simulink model "sim_fake"  (Simulink 8.4)
settings: Solver=ode23s  StartTime=0.0  StopTime=max(time)  FixedStep=0.0001  RelTol=1e-3
values from neighbouring files (symbols this model uses):
  CTRL = ctrl_d(7)    [step4_simulation.m]    (also in step5_yaml.m = ctrl_d(i))
  PLANT = model.chip    [step2_design_controller.m]    (also in step3_check_performance.m = model.combo; step4_simulation.m = model.combo; step99_validation.m = model.combo)
settings Model: Creator=yh3wong  LastModifiedBy=yh3wong
settings DataIOCC: SignalLoggingSaveFormat=Dataset
settings OptimizationCC: ExpressionDepthLimit=128
settings DebuggingCC: UnderspecifiedInitializationDetection=Simplified  MergeDetectMultiDrivingBlocksExec=error  FcnCallInpInsideContextMsg=EnableAllAsError  StateNameClashWarn=none
settings GRTTargetCC: CombineOutputUpdateFcns=on  GRTInterface=off

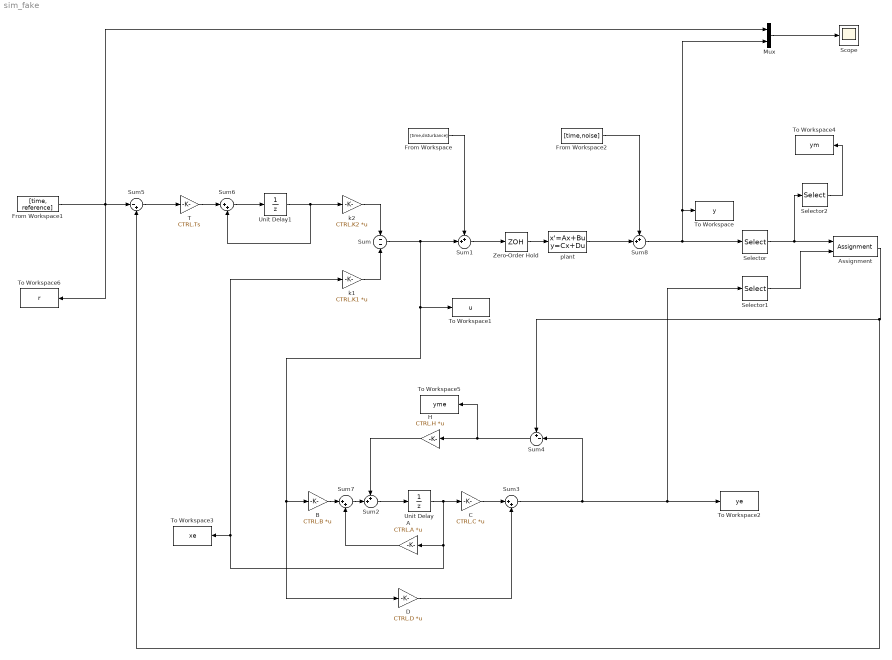
== system sim_fake ==
  A : Gain  Gain=CTRL.A  Multiplication=Matrix(K*u)  SampleTime=CTRL.Ts
  Assignment : Assignment  DiagnosticForDimensions=Warning  SampleTime=CTRL.Ts  Indices=FAKE
  B : Gain  Gain=CTRL.B  Multiplication=Matrix(K*u)  SampleTime=CTRL.Ts
  C : Gain  Gain=CTRL.C  Multiplication=Matrix(K*u)  SampleTime=CTRL.Ts
  D : Gain  Gain=CTRL.D  Multiplication=Matrix(K*u)  SampleTime=CTRL.Ts
  From Workspace : FromWorkspace  VariableName=[time,disturbance]  SampleTime=CTRL.Ts  Interpolate=off  OutputAfterFinalValue=Holding final value
  From Workspace1 : FromWorkspace  VariableName=[time, reference]  SampleTime=CTRL.Ts  Interpolate=off  OutputAfterFinalValue=Holding final value
  From Workspace2 : FromWorkspace  VariableName=[time,noise]  OutputAfterFinalValue=Holding final value
  H : Gain  Gain=CTRL.H  Multiplication=Matrix(K*u)  SampleTime=CTRL.Ts
  Mux : Mux  Inputs=2
  Scope : Scope
      settings: YMin=-150  YMax=200
  Selector : Selector  InputPortWidth=length(PLANT.output)  Indices=CTRL.channel_idx
  Selector1 : Selector  InputPortWidth=length(CTRL.output)  Indices=FAKE
  Selector2 : Selector  InputPortWidth=length(CTRL.output)  Indices=REAL
  Sum : Sum  Inputs=-|-  SampleTime=CTRL.Ts
  Sum1 : Sum  Inputs=++|  SampleTime=CTRL.Ts
  Sum2 : Sum  Inputs=++|  SampleTime=CTRL.Ts
  Sum3 : Sum  Inputs=|++  SampleTime=CTRL.Ts
  Sum4 : Sum  Inputs=+-|  SampleTime=CTRL.Ts
  Sum5 : Sum  Inputs=|-+  SampleTime=CTRL.Ts
  Sum6 : Sum  Inputs=|++  SampleTime=CTRL.Ts
  Sum7 : Sum  Inputs=|++  SampleTime=CTRL.Ts
  Sum8 : Sum  Inputs=++|
  T : Gain  Gain=CTRL.Ts  SampleTime=CTRL.Ts
  To Workspace : ToWorkspace  VariableName=y  SaveFormat=Structure With Time  SampleTime=-1
  To Workspace1 : ToWorkspace  VariableName=u  SaveFormat=Structure With Time  SampleTime=CTRL.Ts
  To Workspace2 : ToWorkspace  VariableName=ye  SaveFormat=Structure With Time  SampleTime=CTRL.Ts
  To Workspace3 : ToWorkspace  VariableName=xe  SaveFormat=Structure With Time  SampleTime=CTRL.Ts
  To Workspace4 : ToWorkspace  VariableName=ym  SaveFormat=Structure With Time  SampleTime=-1
  To Workspace5 : ToWorkspace  VariableName=yme  SaveFormat=Structure With Time  SampleTime=CTRL.Ts
  To Workspace6 : ToWorkspace  VariableName=r  SaveFormat=Structure With Time  SampleTime=CTRL.Ts
  Unit Delay : UnitDelay  SampleTime=CTRL.Ts
  Unit Delay1 : UnitDelay  SampleTime=CTRL.Ts
  Zero-Order Hold : ZeroOrderHold  SampleTime=CTRL.Ts
  "k1 " : Gain  Gain=CTRL.K1  Multiplication=Matrix(K*u)  SampleTime=CTRL.Ts
  k2 : Gain  Gain=CTRL.K2  Multiplication=Matrix(K*u)  SampleTime=CTRL.Ts
  plant : StateSpace  A=PLANT.Ac  B=PLANT.Bc  C=PLANT.Cc  D=PLANT.Dc  X0=0
  wires:
  k2/1 -> Sum/1
  "k1 "/1 -> Sum/2
  Zero-Order Hold/1 -> plant/1
  From Workspace/1 -> Sum1/1
  Sum/1 -> D/1, B/1, To Workspace1/1, Sum1/2
  Sum1/1 -> Zero-Order Hold/1
  Unit Delay/1 -> To Workspace3/1, "k1 "/1, A/1, C/1
  C/1 -> Sum3/1
  D/1 -> Sum3/2
  Sum3/1 -> Sum4/2, Selector1/1, To Workspace2/1
  Selector/1 -> Selector2/1, Assignment/1
  Sum4/1 -> To Workspace5/1, H/1
  H/1 -> Sum2/1
  B/1 -> Sum7/1
  A/1 -> Sum7/2
  Unit Delay1/1 -> k2/1, Sum6/2
  Sum6/1 -> Unit Delay1/1
  T/1 -> Sum6/1
  Sum5/1 -> T/1
  Sum2/1 -> Unit Delay/1
  Sum7/1 -> Sum2/2
  plant/1 -> Sum8/2
  Sum8/1 -> Mux/2, To Workspace/1, Selector/1
  From Workspace2/1 -> Sum8/1
  Assignment/1 -> Sum5/2, Sum4/1
  Selector1/1 -> Assignment/2
  From Workspace1/1 -> To Workspace6/1, Mux/1, Sum5/1
  Mux/1 -> Scope/1
  Selector2/1 -> To Workspace4/1
